simulink model "RLS_1a"  (R2023a)
settings: Solver=ode4  StartTime=0.0  StopTime=40  FixedStep=0.005  RelTol=1e-3
InitFcn:
  | RLS
values from neighbouring files (symbols this model uses):
  K_scheduled = zeros(length(V_op), 2)    [CAL3.m]    (also in CUB.m; DLC2.m; MUS.m; OHZ.m)
  V_op = 5:5:85    [CAL3.m]    (also in CUB.m; DLC2.m; MUS.m; OHZ.m)
  X_track = [linspace(0, runway_length, 200)'; runway_length + R_track * cos(theta_circ(2:end))]    [CAL3.m]    (also in CUB.m = [0; 5000]; DLC2.m = 0:0.1:total_track_length; MUS.m = [0; 2000]; OHZ.m = [0; 2000])
  Y_track = [zeros(200, 1); R_track + R_track * sin(theta_circ(2:end))]    [CAL3.m]    (also in CUB.m = [0; 0]; DLC2.m = zeros(size(X_track)); MUS.m = [0; 0]; OHZ.m = [0; 0])
libraries: simulink x2, slpidlib x1
(part 1 of 2)
settings Model: NumberOfSteps=1000  SnapshotBufferSize=1000  SnapshotInterval=1000  Creator=KBISWAS  LastModifiedBy=KBISWAS

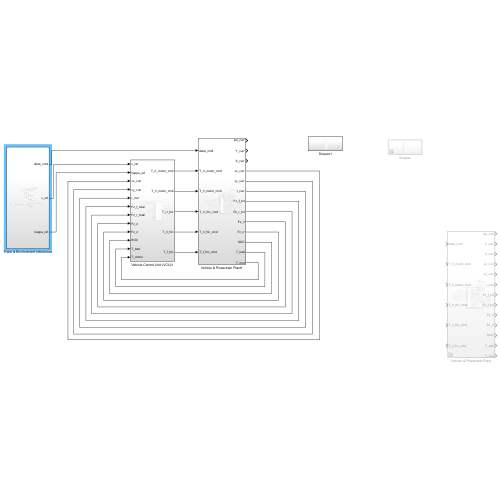
[thumbnail: Simulink's stored preview of the top-level diagram]
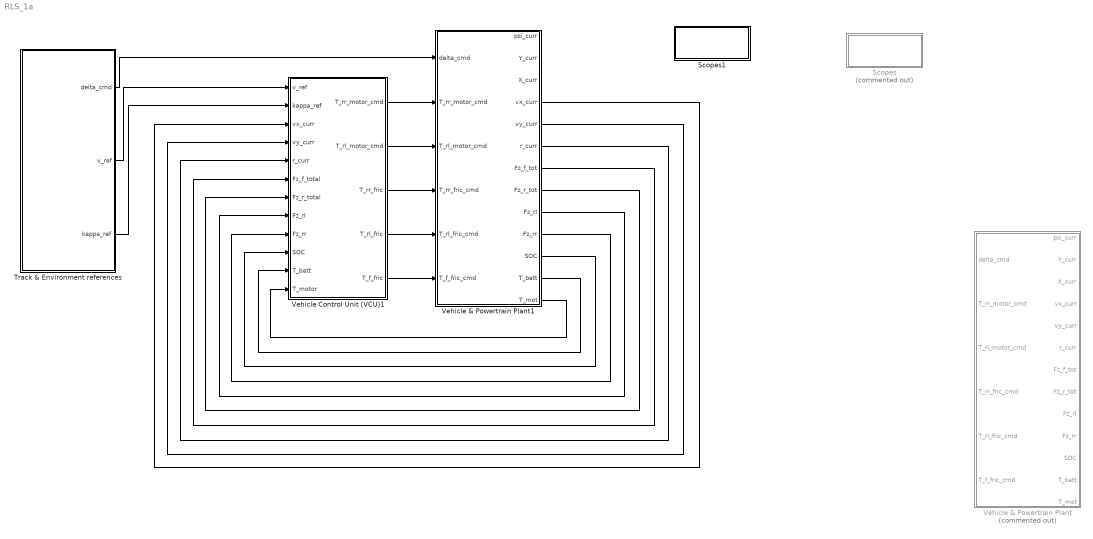
== system RLS_1a ==
  Scopes : Subsystem  Commented=on
  Scopes1 : Subsystem
  Track & Environment references : Subsystem
  Vehicle & Powertrain Plant : Subsystem  Commented=on
  Vehicle & Powertrain Plant1 : Subsystem
  Vehicle Control Unit (VCU)1 : Subsystem
  wires:
  Track & Environment references/2(v_ref) -> Vehicle Control Unit (VCU)1/1(v_ref)
  Vehicle Control Unit (VCU)1/1(T_rr_motor_cmd) -> Vehicle & Powertrain Plant1/2(T_rr_motor_cmd)
  Track & Environment references/3(kappa_ref) -> Vehicle Control Unit (VCU)1/2(kappa_ref)
  Track & Environment references/1(delta_cmd) -> Vehicle & Powertrain Plant1/1(delta_cmd)
  Vehicle Control Unit (VCU)1/2(T_rl_motor_cmd) -> Vehicle & Powertrain Plant1/3(T_rl_motor_cmd)
  Vehicle Control Unit (VCU)1/3(T_rr_fric) -> Vehicle & Powertrain Plant1/4(T_rr_fric_cmd)
  Vehicle Control Unit (VCU)1/4(T_rl_fric) -> Vehicle & Powertrain Plant1/5(T_rl_fric_cmd)
  Vehicle Control Unit (VCU)1/5(T_f_fric) -> Vehicle & Powertrain Plant1/6(T_f_fric_cmd)
  Vehicle & Powertrain Plant1/4(vx_curr) -> Vehicle Control Unit (VCU)1/3(vx_curr)
  Vehicle & Powertrain Plant1/5(vy_curr) -> Vehicle Control Unit (VCU)1/4(vy_curr)
  Vehicle & Powertrain Plant1/6(r_curr) -> Vehicle Control Unit (VCU)1/5(r_curr)
  Vehicle & Powertrain Plant1/7(Fz_f_tot) -> Vehicle Control Unit (VCU)1/6(Fz_f_total)
  Vehicle & Powertrain Plant1/8(Fz_r_tot) -> Vehicle Control Unit (VCU)1/7(Fz_r_total)
  Vehicle & Powertrain Plant1/9(Fz_rl) -> Vehicle Control Unit (VCU)1/8(Fz_rl)
  Vehicle & Powertrain Plant1/10(Fz_rr) -> Vehicle Control Unit (VCU)1/9(Fz_rr)
  Vehicle & Powertrain Plant1/11(SOC) -> Vehicle Control Unit (VCU)1/10(SOC)
  Vehicle & Powertrain Plant1/12(T_batt) -> Vehicle Control Unit (VCU)1/11(T_batt)
  Vehicle & Powertrain Plant1/13(T_mot) -> Vehicle Control Unit (VCU)1/12(T_motor)

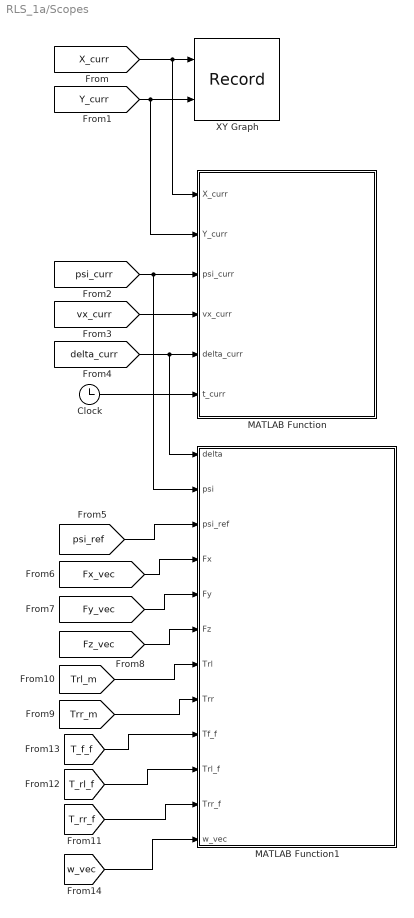
== system RLS_1a/Scopes ==
  Clock : Clock
  MATLAB Function : MATLAB Function  TreatAsAtomicUnit=on
  MATLAB Function1 : MATLAB Function  TreatAsAtomicUnit=on
  XY Graph : Record  FileSettingsInternal="{\"entries\":[{\"content\":{\"excelSettings\":{\"content\":{},\"type\":\"Streamout.ExcelSettings\"}},\"type\":\"Streamout.FileSettingStorage\",\"uuid\":\"\"}],\"packageUris\":[\"http:\\/\\/schema.mathworks.com\\/mf0\\/streamout_blocks\\/R2020a\"],\"version\":\"1.0\"}"  Layout=[1 1]  SignalsInternal="{\"entries\":[{\"content\":{},\"type\":\"RecordBlkView.InputSignals\",\"uuid\":\"\"}],\"packageUris\":[\"http:\\/\\/schema.mathworks.com\\/mf0\\/streamout_blocks\\/R2020a\"],\"version\":\"1.0\"}"  VisualizationBindings="{\"xyplotplugin\":{\"info\":[{\"series\":[],\"subplotID\":1}]}}"  CompatibilityTag=XY
  wires:
  [X_curr] -> MATLAB Function/1(X_curr), XY Graph/1
  [Y_curr] -> MATLAB Function/2(Y_curr), XY Graph/2
  [psi_curr] -> MATLAB Function/3(psi_curr), MATLAB Function1/2(psi)
  [vx_curr] -> MATLAB Function/4(vx_curr)
  [delta_curr] -> MATLAB Function1/1(delta), MATLAB Function/5(delta_curr)
  Clock/1 -> MATLAB Function/6(t_curr)
  [psi_ref] -> MATLAB Function1/3(psi_ref)
  [Fx_vec] -> MATLAB Function1/4(Fx)
  [Fy_vec] -> MATLAB Function1/5(Fy)
  [Fz_vec] -> MATLAB Function1/6(Fz)
  [Trr_m] -> MATLAB Function1/8(Trr)
  [Trl_m] -> MATLAB Function1/7(Trl)
  [T_f_f] -> MATLAB Function1/9(Tf_f)
  [T_rr_f] -> MATLAB Function1/11(Trr_f)
  [T_rl_f] -> MATLAB Function1/10(Trl_f)
  [w_vec] -> MATLAB Function1/12(w_vec)

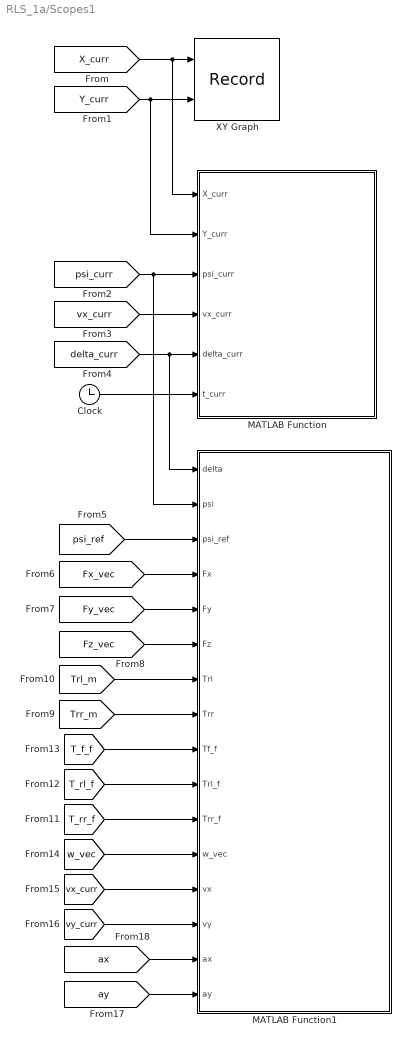
== system RLS_1a/Scopes1 ==
  Clock : Clock
  MATLAB Function : MATLAB Function  TreatAsAtomicUnit=on
  MATLAB Function1 : MATLAB Function  TreatAsAtomicUnit=on
  XY Graph : Record  FileSettingsInternal="{\"entries\":[{\"content\":{\"excelSettings\":{\"content\":{},\"type\":\"Streamout.ExcelSettings\"}},\"type\":\"Streamout.FileSettingStorage\",\"uuid\":\"\"}],\"packageUris\":[\"http:\\/\\/schema.mathworks.com\\/mf0\\/streamout_blocks\\/R2020a\"],\"version\":\"1.0\"}"  Layout=[1 1]  SignalsInternal="{\"entries\":[{\"content\":{\"signals\":[{\"content\":{\"blockPath\":[],\"dimensions\":[1],\"domain\":\"\",\"lineColor\":\"#a2142f\",\"plots\":[1],\"port\":1,\"sid\":[\"\"],\"signalID\":386165,\"signalName\":\"From\"},\"type\":\"RecordBlkView.Signal\",\"uuid\":\"\"},{\"content\":{\"blockPath\":[],\"dimensions\":[1],\"domain\":\"\",\"lineColor\":\"#139fff\",\"plots\":[1],\"port\":2,\"sid\":[\"\"],\"signalID\":386169,\"signalName\":\"From1\"},\"type\":\"RecordBlkView.Signal\",\"uuid\":\"\"}]},\"type\":\"RecordBlkView.InputSignals\",\"uuid\":\"\"}],\"packageUris\":[\"http:\\/\\/schema.mathworks.com\\/mf0\\/streamout_blocks\\/R2020a\"],\"version\":\"1.0\"}"  VisualizationBindings="{\"xyplotplugin\":{\"info\":[{\"series\":[{\"bindingParametersList\":[{\"parameter\":\"X-Axis\",\"signalID\":386165,\"signalName\":\"From\"},{\"parameter\":\"Y-Axis\",\"signalID\":386169,\"signalName\":\"From1\"}],\"seriesID\":29660}],\"subplotID\":1}]}}"  CompatibilityTag=XY
  wires:
  [X_curr] -> MATLAB Function/1(X_curr), XY Graph/1
  [Y_curr] -> MATLAB Function/2(Y_curr), XY Graph/2
  [psi_curr] -> MATLAB Function/3(psi_curr), MATLAB Function1/2(psi)
  [vx_curr] -> MATLAB Function/4(vx_curr)
  [delta_curr] -> MATLAB Function1/1(delta), MATLAB Function/5(delta_curr)
  Clock/1 -> MATLAB Function/6(t_curr)
  [psi_ref] -> MATLAB Function1/3(psi_ref)
  [Fx_vec] -> MATLAB Function1/4(Fx)
  [Fy_vec] -> MATLAB Function1/5(Fy)
  [Fz_vec] -> MATLAB Function1/6(Fz)
  [Trr_m] -> MATLAB Function1/8(Trr)
  [Trl_m] -> MATLAB Function1/7(Trl)
  [T_f_f] -> MATLAB Function1/9(Tf_f)
  [T_rr_f] -> MATLAB Function1/11(Trr_f)
  [T_rl_f] -> MATLAB Function1/10(Trl_f)
  [w_vec] -> MATLAB Function1/12(w_vec)
  [vx_curr] -> MATLAB Function1/13(vx)
  [vy_curr] -> MATLAB Function1/14(vy)
  [ax] -> MATLAB Function1/15(ax)
  [ay] -> MATLAB Function1/16(ay)

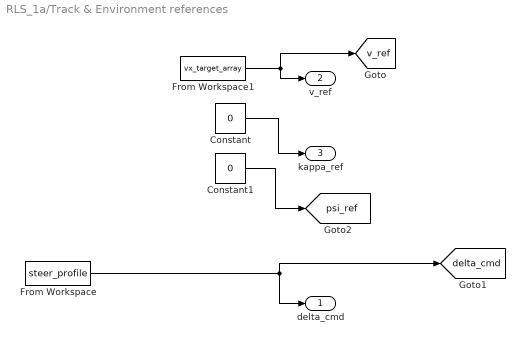
== system RLS_1a/Track & Environment references ==
  Constant : Constant  Value=0
  Constant1 : Constant  Value=0
  From Workspace : FromWorkspace  VariableName=steer_profile
  From Workspace1 : FromWorkspace  VariableName=vx_target_array
  delta_cmd : Outport
  v_ref : Outport  Port=2
  kappa_ref : Outport  Port=3
  tag scope: delta_cmd=global, psi_ref=global, v_ref=global
  wires:
  From Workspace/1 -> [delta_cmd], delta_cmd/1
  From Workspace1/1 -> v_ref/1, [v_ref]
  Constant1/1 -> [psi_ref]
  Constant/1 -> kappa_ref/1

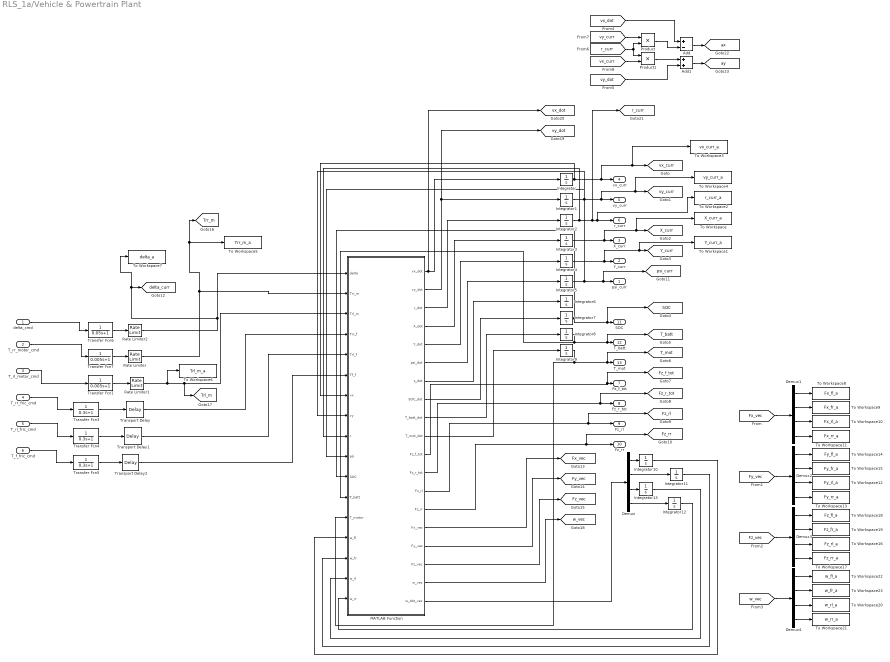
== system RLS_1a/Vehicle & Powertrain Plant ==
  delta_cmd : Inport
  T_rr_motor_cmd : Inport  Port=2
  T_rl_motor_cmd : Inport  Port=3
  T_rr_fric_cmd : Inport  Port=4
  T_rl_fric_cmd : Inport  Port=5
  T_f_fric_cmd : Inport  Port=6
  Add : Sum  Inputs=+-
  Add1 : Sum
  Demux{,1..4} (5 alike) : Demux
  Integrator : Integrator  InitialCondition=5
  Integrator{1..6,10..13} (10 alike) : Integrator
  Integrator7 : Integrator  InitialCondition=0.9
  Integrator8 : Integrator  InitialCondition=30
  Integrator9 : Integrator  InitialCondition=30
  MATLAB Function : MATLAB Function  TreatAsAtomicUnit=on
  Product : Product
  Product1 : Product
  Rate Limiter : RateLimiter  RisingSlewLimit=1500  FallingSlewLimit=-1500  SampleTimeMode=inherited
  Rate Limiter1 : RateLimiter  RisingSlewLimit=1500  FallingSlewLimit=-1500  SampleTimeMode=inherited
  Rate Limiter2 : RateLimiter  RisingSlewLimit=0.05  FallingSlewLimit=-0.05  SampleTimeMode=inherited
  To Workspace : ToWorkspace  VariableName=X_curr_a  SaveFormat=Timeseries  SampleTime=-1
  To Workspace1 : ToWorkspace  VariableName=Y_curr_a  SaveFormat=Timeseries  SampleTime=-1
  To Workspace10 : ToWorkspace  VariableName=Fx_rl_a  SaveFormat=Timeseries  SampleTime=-1
  To Workspace11 : ToWorkspace  VariableName=Fx_rr_a  SaveFormat=Timeseries  SampleTime=-1
  To Workspace12 : ToWorkspace  VariableName=Fy_rl_a  SaveFormat=Timeseries  SampleTime=-1
  To Workspace13 : ToWorkspace  VariableName=Fy_rr_a  SaveFormat=Timeseries  SampleTime=-1
  To Workspace14 : ToWorkspace  VariableName=Fy_fl_a  SaveFormat=Timeseries  SampleTime=-1
  To Workspace15 : ToWorkspace  VariableName=Fy_fr_a  SaveFormat=Timeseries  SampleTime=-1
  To Workspace16 : ToWorkspace  VariableName=Fz_rl_a  SaveFormat=Timeseries  SampleTime=-1
  To Workspace17 : ToWorkspace  VariableName=Fz_rr_a  SaveFormat=Timeseries  SampleTime=-1
  To Workspace18 : ToWorkspace  VariableName=Fz_fl_a  SaveFormat=Timeseries  SampleTime=-1
  To Workspace19 : ToWorkspace  VariableName=Fz_fr_a  SaveFormat=Timeseries  SampleTime=-1
  To Workspace2 : ToWorkspace  VariableName=r_curr_a  SaveFormat=Timeseries  SampleTime=-1
  To Workspace20 : ToWorkspace  VariableName=w_rl_a  SaveFormat=Timeseries  SampleTime=-1
  To Workspace21 : ToWorkspace  VariableName=w_rr_a  SaveFormat=Timeseries  SampleTime=-1
  To Workspace22 : ToWorkspace  VariableName=w_fl_a  SaveFormat=Timeseries  SampleTime=-1
  To Workspace23 : ToWorkspace  VariableName=w_fr_a  SaveFormat=Timeseries  SampleTime=-1
  To Workspace3 : ToWorkspace  VariableName=vx_curr_a  SaveFormat=Timeseries  SampleTime=-1
  To Workspace4 : ToWorkspace  VariableName=vy_curr_a  SaveFormat=Timeseries  SampleTime=-1
  To Workspace5 : ToWorkspace  VariableName=Trr_m_a  SaveFormat=Timeseries  SampleTime=-1
  To Workspace6 : ToWorkspace  VariableName=Trl_m_a  SaveFormat=Timeseries  SampleTime=-1
  To Workspace7 : ToWorkspace  VariableName=delta_a  SaveFormat=Timeseries  SampleTime=-1
  To Workspace8 : ToWorkspace  VariableName=Fx_fl_a  SaveFormat=Timeseries  SampleTime=-1
  To Workspace9 : ToWorkspace  VariableName=Fx_fr_a  SaveFormat=Timeseries  SampleTime=-1
  Transfer Fcn1 : TransferFcn  Denominator=[0.005 1]
  Transfer Fcn3 : TransferFcn  Denominator=[0.3 1]
  Transfer Fcn4 : TransferFcn  Denominator=[0.3 1]
  Transfer Fcn5 : TransferFcn  Denominator=[0.3 1]
  Transfer Fcn6 : TransferFcn  Numerator=1  Denominator=[0.05 1]
  Transfer Fcn7 : TransferFcn  Denominator=[0.005 1]
  Transport Delay : TransportDelay  DelayTime=0.03
  Transport Delay1 : TransportDelay  DelayTime=0.03
  Transport Delay2 : TransportDelay  DelayTime=0.03
  psi_curr : Outport
  Y_curr : Outport  Port=2
  X_curr : Outport  Port=3
  vx_curr : Outport  Port=4
  vy_curr : Outport  Port=5
  r_curr : Outport  Port=6
  Fz_f_tot : Outport  Port=7
  Fz_r_tot : Outport  Port=8
  Fz_rl : Outport  Port=9
  Fz_rr : Outport  Port=10
  SOC : Outport  Port=11
  T_batt : Outport  Port=12
  T_mot : Outport  Port=13
  tag scope: Fx_vec=global, Fy_vec=global, Fz_f_tot=global, Fz_r_tot=global, Fz_rl=global, Fz_rr=global, Fz_vec=global, SOC=global, T_batt=global, T_mot=global, Trl_m=global, Trr_m=global, X_curr=global, Y_curr=global, ax=global, ay=global, delta_curr=global, psi_curr=global, r_curr=global, vx_curr=global, vx_dot=global, vy_curr=global, vy_dot=global, w_vec=global
  wires:
  delta_cmd/1 -> Transfer Fcn6/1
  T_rr_motor_cmd/1 -> Transfer Fcn7/1
  T_rl_motor_cmd/1 -> Transfer Fcn1/1
  T_rr_fric_cmd/1 -> Transfer Fcn3/1
  T_rl_fric_cmd/1 -> Transfer Fcn4/1
  T_f_fric_cmd/1 -> Transfer Fcn5/1
  Rate Limiter2/1 -> MATLAB Function/1(delta), To Workspace7/1, [delta_curr]
  Rate Limiter/1 -> MATLAB Function/2(Trr_m), To Workspace5/1, [Trr_m]
  Rate Limiter1/1 -> To Workspace6/1, MATLAB Function/3(Trl_m), [Trl_m]
  Transport Delay/1 -> MATLAB Function/4(Trr_f)
  Transport Delay1/1 -> MATLAB Function/5(Trl_f)
  Transport Delay2/1 -> MATLAB Function/6(Tf_f)
  MATLAB Function/3(r_dot) -> Integrator2/1
  MATLAB Function/4(X_dot) -> Integrator3/1
  MATLAB Function/5(Y_dot) -> Integrator4/1
  MATLAB Function/6(psi_dot) -> Integrator5/1
  MATLAB Function/7(s_dot) -> Integrator6/1
  MATLAB Function/8(SOC_dot) -> Integrator7/1
  Integrator/1 -> MATLAB Function/7(vx), To Workspace3/1, [vx_curr], vx_curr/1
  Integrator1/1 -> MATLAB Function/8(vy), To Workspace4/1, [vy_curr], vy_curr/1
  Integrator5/1 -> MATLAB Function/10(psi), [psi_curr], psi_curr/1
  Integrator8/1 -> MATLAB Function/12(T_batt), [T_batt], T_batt/1
  Integrator9/1 -> MATLAB Function/13(T_motor), [T_mot], T_mot/1
  Integrator4/1 -> To Workspace1/1, [Y_curr], Y_curr/1
  Integrator3/1 -> To Workspace/1, [X_curr], X_curr/1
  MATLAB Function/11(Fz_f_tot) -> [Fz_f_tot], Fz_f_tot/1
  Integrator7/1 -> MATLAB Function/11(SOC), [SOC], SOC/1
  MATLAB Function/14(Fz_rr) -> [Fz_rr], Fz_rr/1
  MATLAB Function/15(Fx_vec) -> [Fx_vec]
  MATLAB Function/17(Fz_vec) -> [Fz_vec]
  MATLAB Function/9(T_batt_dot) -> Integrator8/1
  MATLAB Function/10(T_mot_dot) -> Integrator9/1
  MATLAB Function/12(Fz_r_tot) -> [Fz_r_tot], Fz_r_tot/1
  MATLAB Function/13(Fz_rl) -> [Fz_rl], Fz_rl/1
  MATLAB Function/16(Fy_vec) -> [Fy_vec]
  MATLAB Function/18(w_vec) -> [w_vec]
  Demux/4 -> Integrator12/1
  Demux/3 -> Integrator13/1
  Demux/2 -> Integrator11/1
  Demux/1 -> Integrator10/1
  MATLAB Function/19(w_dot_vec) -> Demux/1
  Integrator10/1 -> MATLAB Function/14(w_fl)
  Integrator11/1 -> MATLAB Function/15(w_fr)
  Integrator12/1 -> MATLAB Function/17(w_rr)
  Integrator13/1 -> MATLAB Function/16(w_rl)
  Transfer Fcn6/1 -> Rate Limiter2/1
  Transfer Fcn7/1 -> Rate Limiter/1
  Transfer Fcn1/1 -> Rate Limiter1/1
  Transfer Fcn4/1 -> Transport Delay1/1
  Transfer Fcn5/1 -> Transport Delay2/1
  Transfer Fcn3/1 -> Transport Delay/1
  [vx_dot] -> Add/1
  Product/1 -> Add/2
  MATLAB Function/2(vy_dot) -> [vy_dot], Integrator1/1
  Add1/1 -> [ay]
  MATLAB Function/1(vx_dot) -> [vx_dot], Integrator/1
  [vy_curr] -> Product/1
  Integrator2/1 -> [r_curr], To Workspace2/1, r_curr/1, MATLAB Function/9(r)
  [vy_dot] -> Add1/2
  [vx_curr] -> Product1/2
  [r_curr] -> Product1/1, Product/2
  Product1/1 -> Add1/1
  Add/1 -> [ax]
  Demux4/4 -> To Workspace21/1
  Demux4/3 -> To Workspace20/1
  Demux4/1 -> To Workspace22/1
  Demux4/2 -> To Workspace23/1
  [Fy_vec] -> Demux2/1
  [Fz_vec] -> Demux3/1
  [Fx_vec] -> Demux1/1
  Demux3/4 -> To Workspace17/1
  Demux2/2 -> To Workspace15/1
  Demux3/2 -> To Workspace19/1
  Demux3/1 -> To Workspace18/1
  Demux2/1 -> To Workspace14/1
  Demux1/3 -> To Workspace10/1
  Demux1/4 -> To Workspace11/1
  Demux1/2 -> To Workspace9/1
  Demux3/3 -> To Workspace16/1
  Demux2/3 -> To Workspace12/1
  Demux2/4 -> To Workspace13/1
  Demux1/1 -> To Workspace8/1
  [w_vec] -> Demux4/1

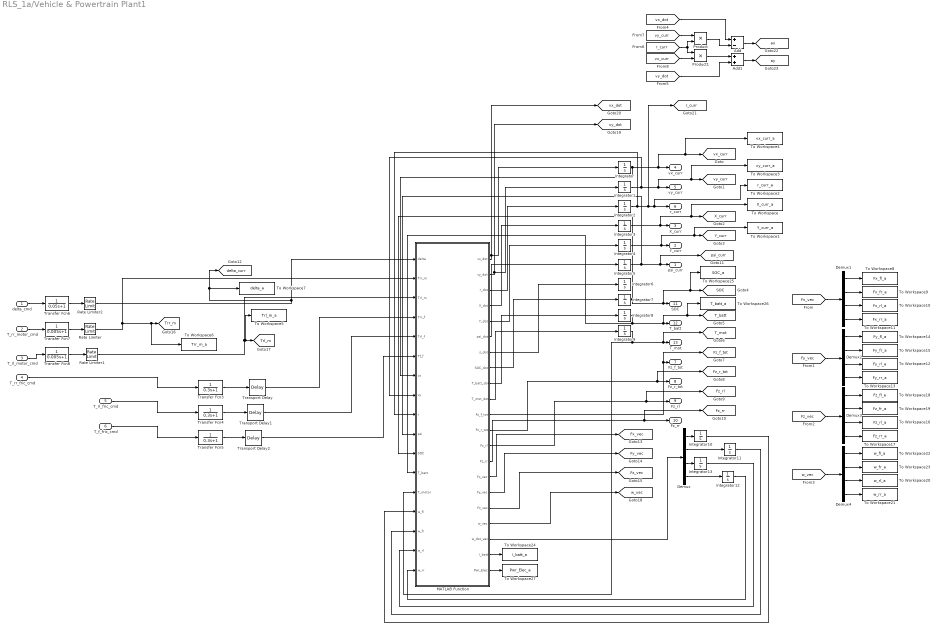
== system RLS_1a/Vehicle & Powertrain Plant1 ==
  delta_cmd : Inport
  T_rr_motor_cmd : Inport  Port=2
  T_rl_motor_cmd : Inport  Port=3
  T_rr_fric_cmd : Inport  Port=4
  T_rl_fric_cmd : Inport  Port=5
  T_f_fric_cmd : Inport  Port=6
  Add : Sum  Inputs=+-
  Add1 : Sum
  Demux{,1..4} (5 alike) : Demux
  Integrator : Integrator  InitialCondition=5
  Integrator{1..6,10..13} (10 alike) : Integrator
  Integrator7 : Integrator  InitialCondition=0.9
  Integrator8 : Integrator  InitialCondition=30
  Integrator9 : Integrator  InitialCondition=30
  MATLAB Function : MATLAB Function  TreatAsAtomicUnit=on
  Product : Product
  Product1 : Product
  Rate Limiter : RateLimiter  RisingSlewLimit=500  FallingSlewLimit=-500  SampleTimeMode=inherited
  Rate Limiter1 : RateLimiter  RisingSlewLimit=500  FallingSlewLimit=-500  SampleTimeMode=inherited
  Rate Limiter2 : RateLimiter  RisingSlewLimit=10  FallingSlewLimit=-10  SampleTimeMode=inherited
  To Workspace : ToWorkspace  VariableName=X_curr_a  SaveFormat=Timeseries  SampleTime=-1
  To Workspace1 : ToWorkspace  VariableName=Y_curr_a  SaveFormat=Timeseries  SampleTime=-1
  To Workspace10 : ToWorkspace  VariableName=Fx_rl_a  SaveFormat=Timeseries  SampleTime=-1
  To Workspace11 : ToWorkspace  VariableName=Fx_rr_a  SaveFormat=Timeseries  SampleTime=-1
  To Workspace12 : ToWorkspace  VariableName=Fy_rl_a  SaveFormat=Timeseries  SampleTime=-1
  To Workspace13 : ToWorkspace  VariableName=Fy_rr_a  SaveFormat=Timeseries  SampleTime=-1
  To Workspace14 : ToWorkspace  VariableName=Fy_fl_a  SaveFormat=Timeseries  SampleTime=-1
  To Workspace15 : ToWorkspace  VariableName=Fy_fr_a  SaveFormat=Timeseries  SampleTime=-1
  To Workspace16 : ToWorkspace  VariableName=Fz_rl_a  SaveFormat=Timeseries  SampleTime=-1
  To Workspace17 : ToWorkspace  VariableName=Fz_rr_a  SaveFormat=Timeseries  SampleTime=-1
  To Workspace18 : ToWorkspace  VariableName=Fz_fl_a  SaveFormat=Timeseries  SampleTime=-1
  To Workspace19 : ToWorkspace  VariableName=Fz_fr_a  SaveFormat=Timeseries  SampleTime=-1
  To Workspace2 : ToWorkspace  VariableName=r_curr_a  SaveFormat=Timeseries  SampleTime=-1
  To Workspace20 : ToWorkspace  VariableName=w_rl_a  SaveFormat=Timeseries  SampleTime=-1
  To Workspace21 : ToWorkspace  VariableName=w_rr_a  SaveFormat=Timeseries  SampleTime=-1
  To Workspace22 : ToWorkspace  VariableName=w_fl_a  SaveFormat=Timeseries  SampleTime=-1
  To Workspace23 : ToWorkspace  VariableName=w_fr_a  SaveFormat=Timeseries  SampleTime=-1
  To Workspace24 : ToWorkspace  VariableName=I_batt_a  SaveFormat=Timeseries  SampleTime=-1
  To Workspace25 : ToWorkspace  VariableName=SOC_a  SaveFormat=Timeseries  SampleTime=-1
  To Workspace26 : ToWorkspace  VariableName=T_batt_a  SaveFormat=Timeseries  SampleTime=-1
  To Workspace27 : ToWorkspace  VariableName=Pwr_Elec_a  SaveFormat=Timeseries  SampleTime=-1
  To Workspace3 : ToWorkspace  VariableName=vy_curr_a  SaveFormat=Timeseries  SampleTime=-1
  To Workspace4 : ToWorkspace  VariableName=vx_curr_a  SaveFormat=Timeseries  SampleTime=-1
  To Workspace5 : ToWorkspace  VariableName=Trl_m_a  SaveFormat=Timeseries  SampleTime=-1
  To Workspace6 : ToWorkspace  VariableName=Trr_m_a  SaveFormat=Timeseries  SampleTime=-1
  To Workspace7 : ToWorkspace  VariableName=delta_a  SaveFormat=Timeseries  SampleTime=-1
  To Workspace8 : ToWorkspace  VariableName=Fx_fl_a  SaveFormat=Timeseries  SampleTime=-1
  To Workspace9 : ToWorkspace  VariableName=Fx_fr_a  SaveFormat=Timeseries  SampleTime=-1
  Transfer Fcn3 : TransferFcn  Denominator=[0.3 1]
  Transfer Fcn4 : TransferFcn  Denominator=[0.3 1]
  Transfer Fcn5 : TransferFcn  Denominator=[0.3 1]
  Transfer Fcn6 : TransferFcn  Numerator=1  Denominator=[0.05 1]
  Transfer Fcn7 : TransferFcn  Denominator=[0.005 1]
  Transfer Fcn8 : TransferFcn  Denominator=[0.005 1]
  Transport Delay : TransportDelay  DelayTime=0.03
  Transport Delay1 : TransportDelay  DelayTime=0.03
  Transport Delay2 : TransportDelay  DelayTime=0.03
  psi_curr : Outport
  Y_curr : Outport  Port=2
  X_curr : Outport  Port=3
  vx_curr : Outport  Port=4
  vy_curr : Outport  Port=5
  r_curr : Outport  Port=6
  Fz_f_tot : Outport  Port=7
  Fz_r_tot : Outport  Port=8
  Fz_rl : Outport  Port=9
  Fz_rr : Outport  Port=10
  SOC : Outport  Port=11
  T_batt : Outport  Port=12
  T_mot : Outport  Port=13
  tag scope: Fx_vec=global, Fy_vec=global, Fz_f_tot=global, Fz_r_tot=global, Fz_rl=global, Fz_rr=global, Fz_vec=global, SOC=global, T_batt=global, T_mot=global, Trl_m=global, Trr_m=global, X_curr=global, Y_curr=global, ax=global, ay=global, delta_curr=global, psi_curr=global, r_curr=global, vx_curr=global, vx_dot=global, vy_curr=global, vy_dot=global, w_vec=global
  wires:
  delta_cmd/1 -> Transfer Fcn6/1
  T_rr_fric_cmd/1 -> Transfer Fcn3/1
  T_rl_fric_cmd/1 -> Transfer Fcn4/1
  T_f_fric_cmd/1 -> Transfer Fcn5/1
  Transfer Fcn6/1 -> Rate Limiter2/1
  Rate Limiter/1 -> MATLAB Function/2(Trr_m), To Workspace6/1, [Trr_m]
  Rate Limiter1/1 -> MATLAB Function/3(Trl_m), To Workspace5/1, [Trl_m]
  Transfer Fcn3/1 -> Transport Delay/1
  Transfer Fcn4/1 -> Transport Delay1/1
  Transfer Fcn5/1 -> Transport Delay2/1
  MATLAB Function/1(vx_dot) -> [vx_dot], Integrator/1
  MATLAB Function/2(vy_dot) -> [vy_dot], Integrator1/1
  MATLAB Function/3(r_dot) -> Integrator2/1
  MATLAB Function/4(X_dot) -> Integrator3/1
  MATLAB Function/5(Y_dot) -> Integrator4/1
  MATLAB Function/6(psi_dot) -> Integrator5/1
  MATLAB Function/7(s_dot) -> Integrator6/1
  MATLAB Function/8(SOC_dot) -> Integrator7/1
  Integrator/1 -> MATLAB Function/7(vx), To Workspace4/1, [vx_curr], vx_curr/1
  Integrator1/1 -> MATLAB Function/8(vy), To Workspace3/1, [vy_curr], vy_curr/1
  Integrator2/1 -> [r_curr], To Workspace2/1, r_curr/1, MATLAB Function/9(r)
  Integrator5/1 -> MATLAB Function/10(psi), [psi_curr], psi_curr/1
  Integrator8/1 -> MATLAB Function/12(T_batt), To Workspace26/1, [T_batt], T_batt/1
  Integrator9/1 -> MATLAB Function/13(T_motor), [T_mot], T_mot/1
  Integrator4/1 -> To Workspace1/1, [Y_curr], Y_curr/1
  Integrator3/1 -> To Workspace/1, [X_curr], X_curr/1
  MATLAB Function/11(Fz_f_tot) -> [Fz_f_tot], Fz_f_tot/1
  Integrator7/1 -> MATLAB Function/11(SOC), To Workspace25/1, [SOC], SOC/1
  MATLAB Function/14(Fz_rr) -> [Fz_rr], Fz_rr/1
  MATLAB Function/15(Fx_vec) -> [Fx_vec]
  MATLAB Function/17(Fz_vec) -> [Fz_vec]
  MATLAB Function/9(T_batt_dot) -> Integrator8/1
  MATLAB Function/10(T_mot_dot) -> Integrator9/1
  MATLAB Function/12(Fz_r_tot) -> [Fz_r_tot], Fz_r_tot/1
  MATLAB Function/13(Fz_rl) -> [Fz_rl], Fz_rl/1
  MATLAB Function/16(Fy_vec) -> [Fy_vec]
  MATLAB Function/18(w_vec) -> [w_vec]
  Demux/4 -> Integrator12/1
  Demux/3 -> Integrator13/1
  Demux/2 -> Integrator11/1
  Demux/1 -> Integrator10/1
  MATLAB Function/19(w_dot_vec) -> Demux/1
  Integrator10/1 -> MATLAB Function/14(w_fl)
  Integrator11/1 -> MATLAB Function/15(w_fr)
  Integrator12/1 -> MATLAB Function/17(w_rr)
  Integrator13/1 -> MATLAB Function/16(w_rl)
  T_rr_motor_cmd/1 -> Transfer Fcn7/1
  Transfer Fcn7/1 -> Rate Limiter/1
  Transfer Fcn8/1 -> Rate Limiter1/1
  T_rl_motor_cmd/1 -> Transfer Fcn8/1
  [Fx_vec] -> Demux1/1
  Demux1/1 -> To Workspace8/1
  Demux1/2 -> To Workspace9/1
  Demux1/3 -> To Workspace10/1
  Demux1/4 -> To Workspace11/1
  Demux2/2 -> To Workspace15/1
  Demux2/4 -> To Workspace13/1
  Demux2/1 -> To Workspace14/1
  [Fy_vec] -> Demux2/1
  Demux2/3 -> To Workspace12/1
  [Fz_vec] -> Demux3/1
  Demux3/1 -> To Workspace18/1
  Demux3/3 -> To Workspace16/1
  Demux3/4 -> To Workspace17/1
  Demux3/2 -> To Workspace19/1
  Demux4/2 -> To Workspace23/1
  Demux4/4 -> To Workspace21/1
  Demux4/1 -> To Workspace22/1
  Demux4/3 -> To Workspace20/1
  [w_vec] -> Demux4/1
  [vy_curr] -> Product/1
  [r_curr] -> Product1/1, Product/2
  Product/1 -> Add/2
  [vx_dot] -> Add/1
  [vx_curr] -> Product1/2
  Product1/1 -> Add1/1
  [vy_dot] -> Add1/2
  Add/1 -> [ax]
  Add1/1 -> [ay]
  MATLAB Function/20(I_batt) -> To Workspace24/1
  MATLAB Function/21(Pwr_Elec) -> To Workspace27/1
  Rate Limiter2/1 -> MATLAB Function/1(delta), To Workspace7/1, [delta_curr]
  Transport Delay/1 -> MATLAB Function/4(Trr_f)
  Transport Delay1/1 -> MATLAB Function/5(Trl_f)
  Transport Delay2/1 -> MATLAB Function/6(Tf_f)

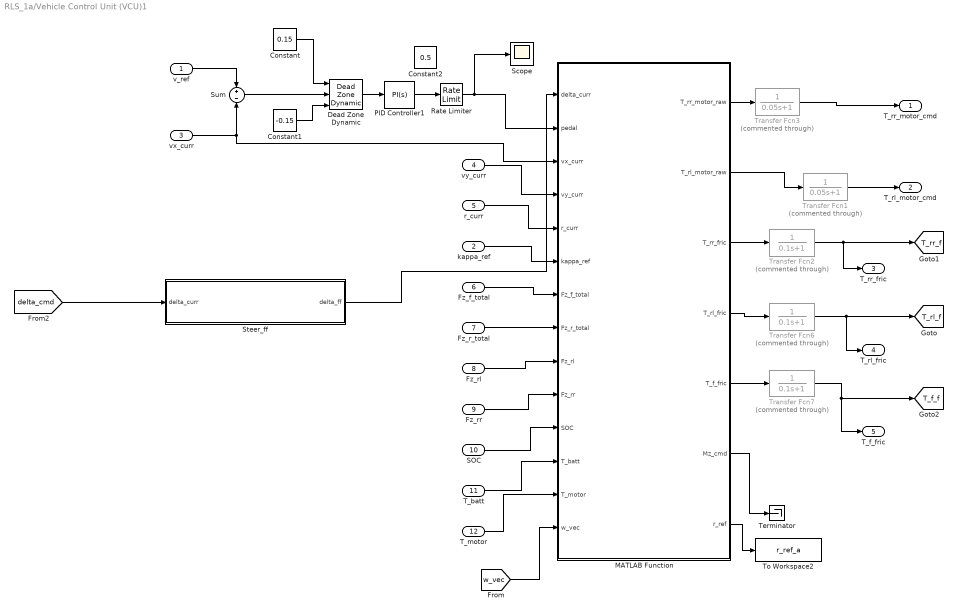
== system RLS_1a/Vehicle Control Unit (VCU)1 ==
  v_ref : Inport
  kappa_ref : Inport  Port=2
  vx_curr : Inport  Port=3
  vy_curr : Inport  Port=4
  r_curr : Inport  Port=5
  Fz_f_total : Inport  Port=6
  Fz_r_total : Inport  Port=7
  Fz_rl : Inport  Port=8
  Fz_rr : Inport  Port=9
  SOC : Inport  Port=10
  T_batt : Inport  Port=11
  T_motor : Inport  Port=12
  Constant : Constant  Value=0.15
  Constant1 : Constant  Value=-0.15
  Constant2 : Constant  Value=0.5
  Dead Zone Dynamic : simulink/Discontinuities/Dead Zone Dynamic
  MATLAB Function : MATLAB Function  TreatAsAtomicUnit=on
  PID Controller1 : slpidlib/PID Controller  Controller=PI  Form=Parallel  TimeDomain=Continuous-time  UseExternalTs=off  SampleTime=-1  IntegratorMethod=Forward Euler  FilterMethod=Forward Euler  ControllerParametersSource=internal  P=0.2  I=0.5  UseKiTs=off  D=0  N=100  UseFilter=on  TunerSelectOption=Transfer Function Based (PID Tuner App)  InitialConditionSource=internal  InitialConditionForIntegrator=0  InitialConditionForFilter=0  DifferentiatorICPrevScaledInput=0  ExternalReset=none  TrackingMode=off  Kt=1  LimitOutput=on  SatLimitsSource=internal  UpperSaturationLimit=1  LowerSaturationLimit=-1  LinearizeAsGain=on  AntiWindupMode=clamping  Kb=1  LimitIntegrator=off  UpperIntegratorSaturationLimit=inf  LowerIntegratorSaturationLimit=-inf  POutMin=[]  POutMax=[]  IOutMin=[]  IOutMax=[]  DOutMin=[]  DOutMax=[]  NOutMin=[]  NOutMax=[]  SumOutMin=[]  SumOutMax=[]  SaturationOutMin=[]  SaturationOutMax=[]  PParamMin=[]  PParamMax=[]  IParamMin=[]  IParamMax=[]  DParamMin=[]  DParamMax=[]  NParamMin=[]  NParamMax=[]  KbParamMin=[]  KbParamMax=[]  KtParamMin=[]  KtParamMax=[]  KbOutMin=[]  KbOutMax=[]  KtOutMin=[]  KtOutMax=[]  IntegratorOutMin=[]  IntegratorOutMax=[]  FilterOutMin=[]  FilterOutMax=[]  SumI1OutMin=[]  SumI1OutMax=[]  SumI2OutMin=[]  SumI2OutMax=[]  SumI3OutMin=[]  SumI3OutMax=[]  SumI4OutMin=[]  SumI4OutMax=[]  SumDOutMin=[]  SumDOutMax=[]  DifferentiatorOutMin=[]  DifferentiatorOutMax=[]  FilterDiffOutCoefMin=[]  FilterDiffOutCoefMax=[]  ReciprocalOutMin=[]  ReciprocalOutMax=[]  SumDenOutMin=[]  SumDenOutMax=[]  SumNumOutMin=[]  SumNumOutMax=[]  DivideOutMin=[]  DivideOutMax=[]  UdiffTsProdOutMin=[]  UdiffTsProdOutMax=[]  NTsProdOutMin=[]  NTsProdOutMax=[]  UintegralTsProdOutMin=[]  UintegralTsProdOutMax=[]  UngainTsProdOutMin=[]  UngainTsProdOutMax=[]  ClampingZeroOutDataTypeStr=Inherit: Inherit via back propagation  ClampingZeroOutMin=[]  ClampingZeroOutMax=[]  FilterDenConstantOutDataTypeStr=Inherit: Inherit via back propagation  FilterDenConstantOutMin=[]  FilterDenConstantOutMax=[]  PCopyOutDataTypeStr=Inherit: Inherit via back propagation  PCopyOutMin=[]  PCopyOutMax=[]  NCopyOutDataTypeStr=Inherit: Inherit via back propagation  NCopyOutMin=[]  NCopyOutMax=[]  IntegratorContinuousStateAttributes=''  IntegratorStateMustResolveToSignalObject=off  IntegratorRTWStateStorageClass=Auto  FilterContinuousStateAttributes=''  FilterStateMustResolveToSignalObject=off  FilterRTWStateStorageClass=Auto  ParallelPVariant=InternalParameters  IdealPVariant=Disabled  IVariant=InternalParameters  DVariant=Disabled  IntegratorVariant=Continuous  SatVariant=Enabled  AWVariant=ContClampingParallel  PCopyVariant=Disabled  TRVariant=Disabled  FdbkBlocksVariant=Forward  IdealPFdbkVariant=Disabled  SatFdbkVariant=Disabled  DerivativeFilterVariant=Disabled  NVariant=Disabled  NCopyVariant=Disabled_SignalSpec  FilterICVariant=Disabled  IntegratorICVariant=InternalICs  ExternalResetVariant=Disabled  TRSumVariant=Passthrough  SumFdbkVariant=Disabled  SumVariant=Sum_PI  TsampFilterVariant=InternalTs  TsampNgainVariant=Passthrough  TsampIntegralVariant=Disabled_SignalSpec  ExternalSaturationOutDataTypeStr=Inherit: Same as second input
  Rate Limiter : RateLimiter  RisingSlewLimit=0.5  FallingSlewLimit=-4  SampleTimeMode=inherited
  Scope : Scope
  Steer_ff : Subsystem
  Sum : Sum  Inputs=+-
  Terminator : Terminator
  To Workspace2 : ToWorkspace  VariableName=r_ref_a  SaveFormat=Timeseries  SampleTime=-1
  Transfer Fcn1 : TransferFcn  Commented=through  Denominator=[0.05 1]
  Transfer Fcn2 : TransferFcn  Commented=through  Denominator=[0.1 1]
  Transfer Fcn3 : TransferFcn  Commented=through  Denominator=[0.05 1]
  Transfer Fcn6 : TransferFcn  Commented=through  Denominator=[0.1 1]
  Transfer Fcn7 : TransferFcn  Commented=through  Denominator=[0.1 1]
  T_rr_motor_cmd : Outport
  T_rl_motor_cmd : Outport  Port=2
  T_rr_fric : Outport  Port=3
  T_rl_fric : Outport  Port=4
  T_f_fric : Outport  Port=5
  tag scope: T_f_f=global, T_rl_f=global, T_rr_f=global
  wires:
  v_ref/1 -> Sum/1
  vy_curr/1 -> MATLAB Function/4(vy_curr)
  r_curr/1 -> MATLAB Function/5(r_curr)
  kappa_ref/1 -> MATLAB Function/6(kappa_ref)
  Fz_f_total/1 -> MATLAB Function/7(Fz_f_total)
  Fz_r_total/1 -> MATLAB Function/8(Fz_r_total)
  Fz_rl/1 -> MATLAB Function/9(Fz_rl)
  Fz_rr/1 -> MATLAB Function/10(Fz_rr)
  SOC/1 -> MATLAB Function/11(SOC)
  T_batt/1 -> MATLAB Function/12(T_batt)
  T_motor/1 -> MATLAB Function/13(T_motor)
  Rate Limiter/1 -> Scope/1, MATLAB Function/2(pedal)
  MATLAB Function/1(T_rr_motor_raw) -> Transfer Fcn3/1
  MATLAB Function/2(T_rl_motor_raw) -> Transfer Fcn1/1
  MATLAB Function/3(T_rr_fric) -> Transfer Fcn2/1
  MATLAB Function/4(T_rl_fric) -> Transfer Fcn6/1
  MATLAB Function/5(T_f_fric) -> Transfer Fcn7/1
  MATLAB Function/6(Mz_cmd) -> Terminator/1
  [w_vec] -> MATLAB Function/14(w_vec)
  MATLAB Function/7(r_ref) -> To Workspace2/1
  Steer_ff/1(delta_ff) -> MATLAB Function/1(delta_curr)
  [delta_cmd] -> Steer_ff/1(delta_curr)
  Transfer Fcn3/1 -> T_rr_motor_cmd/1
  Transfer Fcn1/1 -> T_rl_motor_cmd/1
  Transfer Fcn2/1 -> T_rr_fric/1, [T_rr_f]
  Transfer Fcn6/1 -> T_rl_fric/1, [T_rl_f]
  Transfer Fcn7/1 -> T_f_fric/1, [T_f_f]
  Dead Zone Dynamic/1 -> PID Controller1/1
  Constant/1 -> Dead Zone Dynamic/1
  Sum/1 -> Dead Zone Dynamic/2
  Constant1/1 -> Dead Zone Dynamic/3
  vx_curr/1 -> MATLAB Function/3(vx_curr), Sum/2
  PID Controller1/1 -> Rate Limiter/1

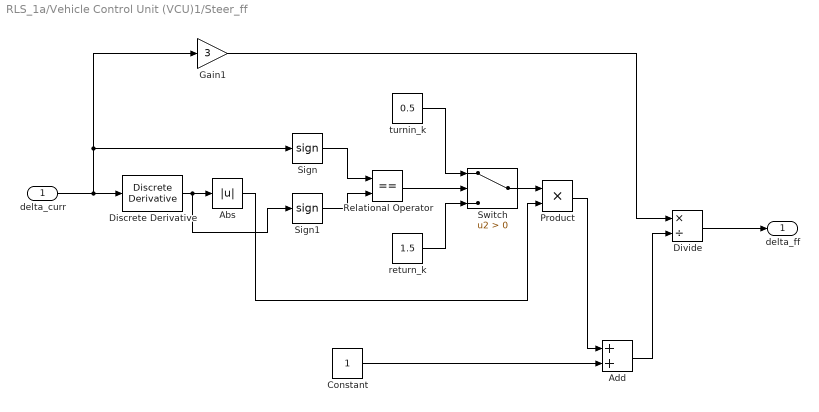
== system RLS_1a/Vehicle Control Unit (VCU)1/Steer_ff ==
  delta_curr : Inport
  Abs : Abs  SaturateOnIntegerOverflow=off
  Add : Sum
  Constant : Constant
  Discrete Derivative : simulink/Discrete/Discrete Derivative  gainval=1.0  ICPrevScaledInput=0.0  OutMin=[]  OutMax=[]  OutDataType=fixdt(1, 16)  OutScaling=2^-10  DoSatur=off
  Divide : Product  Inputs=*/
  Gain1 : Gain  Gain=3
  Product : Product
  Relational Operator : RelationalOperator  Operator===  OutDataTypeStr=boolean  RndMeth=Simplest  InputSameDT=off
  Sign : Signum
  Sign1 : Signum
  Switch : Switch  Criteria=u2 > Threshold  SaturateOnIntegerOverflow=off  InputSameDT=off
  return_k : Constant  Value=1.5
  turnin_k : Constant  Value=0.5
  delta_ff : Outport
  wires:
  Gain1/1 -> Divide/1
  return_k/1 -> Switch/3
  Switch/1 -> Product/1
  Product/1 -> Add/1
  Sign/1 -> Relational Operator/1
  delta_curr/1 -> Discrete Derivative/1, Gain1/1, Sign/1
  Relational Operator/1 -> Switch/2
  Add/1 -> Divide/2
  Discrete Derivative/1 -> Sign1/1, Abs/1
  Abs/1 -> Product/2
  Constant/1 -> Add/2
  Sign1/1 -> Relational Operator/2
  Divide/1 -> delta_ff/1
  turnin_k/1 -> Switch/1

== matlab function RLS_1a/Vehicle & Powertrain Plant/MATLAB Function ==
  data: delta input; Trr_m input; Trl_m input; Trr_f input; Trl_f input; Tf_f input; vx input; vy input; r input; psi input; SOC input; T_batt input; T_motor input; w_fl input; w_fr input; w_rl input; w_rr input; vx_dot output; vy_dot output; r_dot output; X_dot output; Y_dot output; psi_dot output; s_dot output; SOC_dot output; T_batt_dot output; T_mot_dot output; Fz_f_tot output; Fz_r_tot output; Fz_rl output; Fz_rr output; Fx_vec output; Fy_vec output; Fz_vec output; w_vec output; w_dot_vec output; veh_params parameter
function [vx_dot, vy_dot, r_dot, X_dot, Y_dot, psi_dot, s_dot, SOC_dot, T_batt_dot, T_mot_dot, Fz_f_tot, Fz_r_tot, Fz_rl, Fz_rr, Fx_vec, Fy_vec, Fz_vec, w_vec, w_dot_vec] = vehicle_physics_engine(delta, Trr_m, Trl_m, Trr_f, Trl_f, Tf_f, vx, vy, r, psi, SOC, T_batt, T_motor, w_fl, w_fr, w_rl, w_rr, veh_params)
    % =========================================================================
    % STABLE BASELINE 7-DOF PLANAR PHYSICS (Zero Roll/Pitch Delay)
    % =========================================================================
    
    % 1. UNPACK PARAMETERS
    m = veh_params.m; Iz = veh_params.Iz; lf = veh_params.lf; lr = veh_params.lr; L = veh_params.L;
    tw = veh_params.tw; h_cg = veh_params.h_cg; Rw = veh_params.Rw; Iw = veh_params.Iw; 
    G = veh_params.G; g = veh_params.g; rho = veh_params.rho; CdA = veh_params.CdA;
    roll_bias_f = veh_params.roll_bias_f; mu_max = veh_params.mu_max; C_rr = veh_params.C_rr;
    ks_f = veh_params.ks_f; ks_r = veh_params.ks_r; C_tire = veh_params.C_tire; E_tire = veh_params.E_tire;
    
    if abs(vx) < 0.5, vx_safe = 0.5 * sign(vx + 1e-6); else, vx_safe = vx; end
    F_aero_drag = 0.5 * rho * CdA * vx_safe * abs(vx_safe);

    % ---------------------------------------------------------------------
    % 2. INSTANTANEOUS WEIGHT TRANSFER (QUASI-STATIC)
    % ---------------------------------------------------------------------
    Fx_total_tq = (Trr_m + Trl_m)*G + Trr_f + Trl_f + Tf_f;
    ax_inst = (Fx_total_tq/Rw - F_aero_drag) / m;
    ay_inst = vx_safe * r;
    
    dFz_x = m * ax_inst * (h_cg / L);
    dFz_y = m * ay_inst * (h_cg / tw);
    
    Fz_f_tot = m * g * (lr / L) - dFz_x;
    Fz_r_tot = m * g * (lf / L) + dFz_x;
    
    % Instant distribution based on static roll bias
    Fz_fl = max(100, Fz_f_tot/2 - dFz_y * roll_bias_f);
    Fz_fr = max(100, Fz_f_tot/2 + dFz_y * roll_bias_f);
    Fz_rl = max(100, Fz_r_tot/2 - dFz_y * (1 - roll_bias_f));
    Fz_rr = max(100, Fz_r_tot/2 + dFz_y * (1 - roll_bias_f));
    Fz_vec = [Fz_fl, Fz_fr, Fz_rl, Fz_rr];
    
    % ---------------------------------------------------------------------
    % 3. PACEJKA COMBINED SLIP
    % ---------------------------------------------------------------------
    B_f = ks_f / (C_tire * mu_max * (Fz_f_tot/2 + 1e-6)); 
    B_r = ks_r / (C_tire * mu_max * (Fz_r_tot/2 + 1e-6)); 
    
    v_hub_fl = vx_safe - (tw / 2) * r; v_hub_fr = vx_safe + (tw / 2) * r;
    v_hub_rl = vx_safe - (tw / 2) * r; v_hub_rr = vx_safe + (tw / 2) * r;
    
    k_fl = (w_fl * Rw - v_hub_fl) / max(abs(v_hub_fl), 1.0);
    k_fr = (w_fr * Rw - v_hub_fr) / max(abs(v_hub_fr), 1.0);
    k_rl = (w_rl * Rw - v_hub_rl) / max(abs(v_hub_rl), 1.0);
    k_rr = (w_rr * Rw - v_hub_rr) / max(abs(v_hub_rr), 1.0);
    
    alpha_fl = delta - atan((vy + lf * r) / max(abs(v_hub_fl), 1.0));
    alpha_fr = delta - atan((vy + lf * r) / max(abs(v_hub_fr), 1.0));
    alpha_rl = -atan((vy - lr * r) / max(abs(v_hub_rl), 1.0));
    alpha_rr = -atan((vy - lr * r) / max(abs(v_hub_rr), 1.0));
    
    sigma_fl = sqrt(k_fl^2 + tan(alpha_fl)^2) + 1e-6;
    sigma_fr = sqrt(k_fr^2 + tan(alpha_fr)^2) + 1e-6;
    sigma_rl = sqrt(k_rl^2 + tan(alpha_rl)^2) + 1e-6;
    sigma_rr = sqrt(k_rr^2 + tan(alpha_rr)^2) + 1e-6;
    
    F_tot_fl = mu_max * Fz_fl * sin(C_tire * atan(B_f * sigma_fl - E_tire * (B_f * sigma_fl - atan(B_f * sigma_fl))));
    F_tot_fr = mu_max * Fz_fr * sin(C_tire * atan(B_f * sigma_fr - E_tire * (B_f * sigma_fr - atan(B_f * sigma_fr))));
    F_tot_rl = mu_max * Fz_rl * sin(C_tire * atan(B_r * sigma_rl - E_tire * (B_r * sigma_rl - atan(B_r * sigma_rl))));
    F_tot_rr = mu_max * Fz_rr * sin(C_tire * atan(B_r * sigma_rr - E_tire * (B_r * sigma_rr - atan(B_r * sigma_rr))));
    
    Fx_fl = F_tot_fl * (k_fl / sigma_fl) - C_rr * Fz_fl * tanh(v_hub_fl * 10);
    Fx_fr = F_tot_fr * (k_fr / sigma_fr) - C_rr * Fz_fr * tanh(v_hub_fr * 10);
    Fx_rl = F_tot_rl * (k_rl / sigma_rl) - C_rr * Fz_rl * tanh(v_hub_rl * 10);
    Fx_rr = F_tot_rr * (k_rr / sigma_rr) - C_rr * Fz_rr * tanh(v_hub_rr * 10);
    Fx_vec = [Fx_fl, Fx_fr, Fx_rl, Fx_rr];
    
    Fy_fl = F_tot_fl * (tan(alpha_fl) / sigma_fl);
    Fy_fr = F_tot_fr * (tan(alpha_fr) / sigma_fr);
    Fy_rl = F_tot_rl * (tan(alpha_rl) / sigma_rl);
    Fy_rr = F_tot_rr * (tan(alpha_rr) / sigma_rr);
    Fy_vec = [Fy_fl, Fy_fr, Fy_rl, Fy_rr];
    
    % 4. CHASSIS INTEGRATORS
    w_fl_dot = (-abs(Tf_f/2)*sign(w_fl) - Fx_fl*Rw)/Iw;
    w_fr_dot = (-abs(Tf_f/2)*sign(w_fr) - Fx_fr*Rw)/Iw;
    w_rl_dot = (Trl_m*G - abs(Trl_f)*sign(w_rl) - Fx_rl*Rw)/Iw;
    w_rr_dot = (Trr_m*G - abs(Trr_f)*sign(w_rr) - Fx_rr*Rw)/Iw;
    w_dot_vec = [w_fl_dot, w_fr_dot, w_rl_dot, w_rr_dot];
    w_vec = [w_fl, w_fr, w_rl, w_rr];
    
    sum_Fx = (Fx_fl + Fx_fr)*cos(delta) - (Fy_fl + Fy_fr)*sin(delta) + Fx_rl + Fx_rr;
    vx_dot = (sum_Fx - F_aero_drag)/m + vy*r;
    sum_Fy = (Fy_fl + Fy_fr)*cos(delta) + (Fx_fl + Fx_fr)*sin(delta) + Fy_rl + Fy_rr;
    vy_dot = sum_Fy/m - vx_safe*r;
    
    r_dot = (lf*((Fy_fl + Fy_fr)*cos(delta) + (Fx_fl + Fx_fr)*sin(delta)) - lr*(Fy_rl + Fy_rr) + (Fx_rr - Fx_rl)*(tw/2))/Iz;
    
    X_dot = vx_safe*cos(psi) - vy*sin(psi);
    Y_dot = vx_safe*sin(psi) + vy*cos(psi);
    psi_dot = r; s_dot = vx_safe;
    
    % THERMALS & SOC (Simplified Baseline)
    P_mech = (Trr_m + Trl_m)*G*(vx_safe/Rw);
    I_curr = (P_mech / 0.90) / veh_params.V_pack;
    SOC_dot = -I_curr/(veh_params.Cap_Ah*3600);
    T_batt_dot = ((I_curr^2)*veh_params.R_pack - veh_params.hA_cool_batt*(T_batt-veh_params.T_coolant_batt))/(veh_params.m_batt*veh_params.cp_batt);
    T_mot_dot  = (abs(P_mech*0.1) - veh_params.hA_cool_motor*(T_motor-veh_params.T_ambient))/(veh_params.m_motor*veh_params.cp_motor);
end

== matlab function RLS_1a/Scopes/MATLAB Function ==
  settings: updateMethod=DISCRETE
  data: X_curr input; Y_curr input; psi_curr input; vx_curr input; delta_curr input; t_curr input; X_track parameter; Y_track parameter
function live_track_plotter(X_curr, Y_curr, psi_curr, vx_curr, delta_curr, t_curr, X_track, Y_track)
    coder.extrinsic('figure', 'plot', 'hold', 'axis', 'title', 'xlabel', 'ylabel', 'set', 'drawnow', 'animatedline', 'addpoints', 'legend', 'grid', 'patch', 'text');
    
    persistent hFig hCar hTrail hText counter 
    persistent hTimer1 hTimer2 hTimer3 hTimer4 hTimer5
    persistent lap_count lap_start_time lap_trigger_ready
    persistent past_lap_1 past_lap_2 past_lap_3 past_lap_4 past_lap_5
    
    if isempty(counter)
        counter = 0;
        lap_count = 1;
        lap_start_time = 0;
        lap_trigger_ready = false;
        
        past_lap_1 = 0; past_lap_2 = 0; past_lap_3 = 0; past_lap_4 = 0; past_lap_5 = 0;
        
        hFig = figure('Name', 'Live Telemetry: Silverstone / DLC', 'Color', 'w', 'Position', [100, 100, 800, 600]);
        plot(X_track, Y_track, '--', 'Color', [0.4 0.4 0.4], 'LineWidth', 1.5); hold on;
        
        plot(X_track(1), Y_track(1), 'ko', 'MarkerSize', 10, 'MarkerFaceColor', 'g', 'LineWidth', 1.5);
        text(X_track(1) - 50, Y_track(1) + 70, 'Start / Finish', 'FontSize', 10, 'FontWeight', 'bold', 'Color', 'k', 'BackgroundColor', [1 1 1 0.7]);
        
        hTrail = animatedline('Color', 'b', 'LineWidth', 1.5);
        
        hCar = patch(0, 0, [0.8 0 0], 'EdgeColor', 'k', 'LineWidth', 1);
        set(hCar, 'FaceAlpha', 0.8); 
        
        hText = text(0, 0, ' Init...', 'FontSize', 10, 'FontWeight', 'bold', 'BackgroundColor', [1 1 1 0.8], 'EdgeColor', 'k', 'Margin', 2);
        
        box_props = {'Units', 'normalized', 'HorizontalAlignment', 'right', 'FontSize', 12, 'FontWeight', 'bold', 'BackgroundColor', [1 1 1 0.9], 'EdgeColor', 'k', 'Margin', 4, 'Visible', 'off'};
        
        hTimer1 = text(0.95, 0.95, '', box_props{:});
        hTimer2 = text(0.95, 0.89, '', box_props{:});
        hTimer3 = text(0.95, 0.83, '', box_props{:});
        hTimer4 = text(0.95, 0.77, '', box_props{:});
        hTimer5 = text(0.95, 0.71, '', box_props{:});
        
        axis equal; grid on;
        title('Live Vehicle Tracking with Telemetry');
        xlabel('X Position (meters)'); ylabel('Y Position (meters)');
        legend('Reference Track', 'Start/Finish', 'Driven Path', 'EV Position & Heading', 'Telemetry', 'Location', 'best');
    end
    counter = counter + 1;
    
    dist_to_origin = sqrt((X_curr - X_track(1))^2 + (Y_curr - Y_track(1))^2);
    
    if dist_to_origin > 50
        lap_trigger_ready = true;
    end
    
    if lap_trigger_ready && dist_to_origin < 15
        completed_lap_time = t_curr - lap_start_time;
        if lap_count == 1
            past_lap_1 = completed_lap_time;
        elseif lap_count == 2
            past_lap_2 = completed_lap_time;
        elseif lap_count == 3
            past_lap_3 = completed_lap_time;
        elseif lap_count == 4
            past_lap_4 = completed_lap_time;
        elseif lap_count == 5
            past_lap_5 = completed_lap_time;
        end
        
        lap_count = lap_count + 1;
        lap_start_time = t_curr;
        lap_trigger_ready = false; 
    end
    
    if mod(counter, 10) == 0
        addpoints(hTrail, X_curr, Y_curr);
        
        % --- REALISTIC 1:1 VEHICLE SCALING ---
        L_vis = 4.5; % 4.5 meters long
        W_vis = 1.9; % 1.9 meters wide
        % ------------------------------------
        
        base_X = [L_vis/2,  L_vis*0.3,   0,       -L_vis*0.35, -L_vis/2,  -L_vis/2,   -L_vis*0.35,  0,        L_vis*0.3,   L_vis/2];
        base_Y = [0,        W_vis*0.45, W_vis/2,  W_vis/2,     W_vis*0.3, -W_vis*0.3, -W_vis/2,    -W_vis/2, -W_vis*0.45, 0];
        
        R = [cos(psi_curr), -sin(psi_curr); 
             sin(psi_curr),  cos(psi_curr)];
             
        rotated_coords = R * [base_X; base_Y];
        final_X = rotated_coords(1, :) + X_curr;
        final_Y = rotated_coords(2, :) + Y_curr;
        
        set(hCar, 'XData', final_X, 'YData', final_Y);
        
        speed_kmh = vx_curr * 3.6;
        steer_deg = delta_curr * (180 / pi);
        
        telemetry_str = sprintf(' Spd: %.1f km/h\n Steer. Ang.: %.1f deg', speed_kmh, steer_deg);
        
        % Brought the text box much closer to the scaled vehicle
        set(hText, 'Position', [X_curr + 10, Y_curr + 10], 'String', telemetry_str);
        
        current_live_time = t_curr - lap_start_time;
        
        if lap_count == 1
            set(hTimer1, 'String', sprintf(' Lap 1: %d:%06.3f (Live) ', int32(floor(current_live_time/60)), mod(current_live_time, 60)), 'Visible', 'on');
        elseif lap_count > 1
            set(hTimer1, 'String', sprintf(' Lap 1: %d:%06.3f ', int32(floor(past_lap_1/60)), mod(past_lap_1, 60)), 'Visible', 'on');
        end
        
        if lap_count == 2
            set(hTimer2, 'String', sprintf(' Lap 2: %d:%06.3f (Live) ', int32(floor(current_live_time/60)), mod(current_live_time, 60)), 'Visible', 'on');
        elseif lap_count > 2
            set(hTimer2, 'String', sprintf(' Lap 2: %d:%06.3f ', int32(floor(past_lap_2/60)), mod(past_lap_2, 60)), 'Visible', 'on');
        end
        
        if lap_count == 3
            set(hTimer3, 'String', sprintf(' Lap 3: %d:%06.3f (Live) ', int32(floor(current_live_time/60)), mod(current_live_time, 60)), 'Visible', 'on');
        elseif lap_count > 3
            set(hTimer3, 'String', sprintf(' Lap 3: %d:%06.3f ', int32(floor(past_lap_3/60)), mod(past_lap_3, 60)), 'Visible', 'on');
        end
        
        if lap_count == 4
            set(hTimer4, 'String', sprintf(' Lap 4: %d:%06.3f (Live) ', int32(floor(current_live_time/60)), mod(current_live_time, 60)), 'Visible', 'on');
        elseif lap_count > 4
            set(hTimer4, 'String', sprintf(' Lap 4: %d:%06.3f ', int32(floor(past_lap_4/60)), mod(past_lap_4, 60)), 'Visible', 'on');
        end
        
        if lap_count == 5
            set(hTimer5, 'String', sprintf(' Lap 5: %d:%06.3f (Live) ', int32(floor(current_live_time/60)), mod(current_live_time, 60)), 'Visible', 'on');
        elseif lap_count > 5
            set(hTimer5, 'String', sprintf(' Lap 5: %d:%06.3f ', int32(floor(past_lap_5/60)), mod(past_lap_5, 60)), 'Visible', 'on');
        end
        
        drawnow limitrate; 
    end
end

== matlab function RLS_1a/Scopes/MATLAB Function1 ==
  settings: updateMethod=DISCRETE
  data: delta input; psi input; psi_ref input; Fx input; Fy input; Fz input; Trl input; Trr input; Tf_f input; Trl_f input; Trr_f input; w_vec input
function vehicle_frame_plotter(delta, psi, psi_ref, Fx, Fy, Fz, Trl, Trr, Tf_f, Trl_f, Trr_f, w_vec)
    coder.extrinsic('figure', 'plot', 'hold', 'axis', 'title', 'set', 'drawnow', 'patch', 'text', 'line', 'quiver', 'sprintf');
    
    persistent hFig hWheels hSteer hSpokes hPsiRef hPsiAct hFlags hTqFlags hMotors hAxle hCircles hGdots hSwLabel hRwLabel counter
    
    if isempty(counter)
        counter = 0;
        hWheels = zeros(1,4); hFlags = zeros(1,4); hTqFlags = zeros(1,2);
        hMotors = zeros(1,2); hSpokes = zeros(1,3); hCircles = zeros(1,4); hGdots = zeros(1,4);
        hSwLabel = 0.0; hRwLabel = 0.0;
        
        hFig = figure('Name', 'Vehicle Frame Telemetry', 'Color', 'w', 'Position', [950, 100, 750, 750]);
        hold on;
        
        plot([-1, 1, 1, -1, -1], [2, 2, -2, -2, 2], 'k', 'LineWidth', 2);
        hAxle = line([1, -1], [1.5, 1.5], 'Color', [0.2 0.2 0.2], 'LineWidth', 2);
        
        wheel_base = [-.2, .2, .2, -.2]; wheel_wid = [.4, .4, -.4, -.4];
        for i = 1:4; hWheels(i) = double(patch(0, 0, [0.3 0.3 0.3])); end
        
        m_b = [-.15, .15, .15, -.15]; m_w = [.2, .2, -.2, -.2];
        hMotors(1) = double(patch(m_b + 0.6, m_w - 1.5, [0.5 0.5 0.5]));
        hMotors(2) = double(patch(m_b - 0.6, m_w - 1.5, [0.5 0.5 0.5]));
        
        th_c = 0:0.1:2*pi;
        circle_x = cos(th_c); circle_y = sin(th_c);
        c_pos = [2.0, 2.3; -2.0, 2.3; 2.0, -2.3; -2.0, -2.3];
        for i = 1:4
            hCircles(i) = double(plot(c_pos(i,1) + 0.5*circle_x, c_pos(i,2) + 0.5*circle_y, 'Color', [0.6 0 0.6], 'LineStyle', '--', 'LineWidth', 1.2));
            hGdots(i) = double(plot(c_pos(i,1), c_pos(i,2), 'mo', 'MarkerFaceColor', 'm', 'MarkerSize', 5));
        end
        
        th = 0:0.1:2*pi;
        hSteer = double(plot(0.4*cos(th), 0.4*sin(th) + 0.5, 'k', 'LineWidth', 3));
        hSpokes(1) = double(line([0, 0], [0.5, 0.5], 'Color', 'k', 'LineWidth', 2.5));
        hSpokes(2) = double(line([0, 0], [0.5, 0.5], 'Color', 'k', 'LineWidth', 2.5));
        hSpokes(3) = double(line([0, 0], [0.5, 0.5], 'Color', 'k', 'LineWidth', 2.5));
        
        hPsiRef = double(quiver(0, 1.8, 0, 0.8, 'r', 'LineWidth', 2.5, 'MaxHeadSize', 2));
        hPsiAct = double(quiver(0, 1.8, 0, 0.8, 'b', 'LineWidth', 2.5, 'MaxHeadSize', 2));
        
        for i = 1:4; hFlags(i) = double(text(0, 0, '', 'FontSize', 8, 'BackgroundColor', [1 1 1 0.8], 'EdgeColor', 'k')); end
        hTqFlags(1) = double(text(0.6, -1.1, '', 'FontSize', 8, 'FontWeight', 'bold', 'HorizontalAlignment', 'center'));
        hTqFlags(2) = double(text(-0.6, -1.1, '', 'FontSize', 8, 'FontWeight', 'bold', 'HorizontalAlignment', 'center'));
        
        hSwLabel = double(text(0, 0, '', 'FontSize', 9, 'FontWeight', 'bold', 'HorizontalAlignment', 'center'));
        hRwLabel = double(text(0, 2.3, '', 'FontSize', 9, 'FontWeight', 'bold', 'HorizontalAlignment', 'center', 'Color', [0 0.5 0]));
        
        axis([-4.5 4.5 -4.5 4.5]); axis equal; grid on;
        title('Dynamics: Forces, Steering & Friction Circles');
    end
    counter = counter + 1;
    if mod(counter, 10) == 0
        R_delta = [cos(delta) -sin(delta); sin(delta) cos(delta)];
        w_orig = [-.2 .2 .2 -.2; .4 .4 -.4 -.4]; 
        w_rot = R_delta * w_orig;
        
        set(hWheels(1), 'XData', w_rot(1,:) + 1, 'YData', w_rot(2,:) + 1.5);
        set(hWheels(2), 'XData', w_rot(1,:) - 1, 'YData', w_rot(2,:) + 1.5);
        set(hWheels(3), 'XData', w_orig(1,:) + 1, 'YData', w_orig(2,:) - 1.5);
        set(hWheels(4), 'XData', w_orig(1,:) - 1, 'YData', w_orig(2,:) - 1.5);
        
        set(hAxle, 'XData', [mean(w_rot(1,:) + 1), mean(w_rot(1,:) - 1)], 'YData', [mean(w_rot(2,:) + 1.5), mean(w_rot(2,:) + 1.5)]);
        
        sw_a = delta * 14; 
        th_sw = (0:0.1:2*pi) + sw_a;
        set(hSteer, 'XData', 0.4*cos(th_sw), 'YData', 0.4*sin(th_sw) + 0.5);
        
        spk = [0, pi, 1.5*pi] + sw_a;
        for j=1:3; set(hSpokes(j), 'XData', [0, 0.4*cos(spk(j))], 'YData', [0.5, 0.5 + 0.4*sin(spk(j))]); end
        
        set(hSwLabel, 'Position', [0, 0.5], 'String', sprintf('SW: %.1f deg', sw_a * 180/pi));
        set(hRwLabel, 'String', sprintf('RW: %.1f deg', delta * 180/pi));
        
        psi_e = psi_ref - psi; 
        set(hPsiRef, 'UData', 0.8*sin(psi_e), 'VData', 0.8*cos(psi_e));
        set(hPsiAct, 'UData', 0, 'VData', 0.8);
        
        fb = [abs(Tf_f/2), abs(Tf_f/2), abs(Trl_f), abs(Trr_f)]; mu = 1.0;
        c_pos = [2.0, 2.3; -2.0, 2.3; 2.0, -2.3; -2.0, -2.3];
        th_c = 0:0.1:2*pi;
        
        % Convert rad/s to RPM
        rpm_vec = w_vec * (30 / pi);
        
        for i = 1:4
            if fb(i) > 5; set(hWheels(i), 'FaceColor', [0.8 0 0]); else set(hWheels(i), 'FaceColor', [0.3 0.3 0.3]); end
            F_max = max(100, mu * Fz(i));
            scale = 0.5 / 6000; 
            set(hCircles(i), 'XData', c_pos(i,1) + F_max*scale*cos(th_c), 'YData', c_pos(i,2) + F_max*scale*sin(th_c));
            set(hGdots(i), 'XData', c_pos(i,1) + Fy(i)*scale, 'YData', c_pos(i,2) + Fx(i)*scale);
        end
        
        mt = [Trl, Trr];
        for k = 1:2
            if mt(k) > 0.1; set(hMotors(k), 'FaceColor', [0 0.7 0]); elseif mt(k) < -0.1; set(hMotors(k), 'FaceColor', [0.7 0 0]); else set(hMotors(k), 'FaceColor', [0.5 0.5 0.5]); end
            set(hTqFlags(k), 'String', sprintf('Mot. Trq.\n%.1f Nm', mt(k)));
        end
        
        pos = [2.8, 1.5; -4.1, 1.5; 2.8, -1.5; -4.1, -1.5];
        for i = 1:4
            f_str = sprintf('Fx: %.0f\nFy: %.0f\nFz: %.0f\nFric: %.1f\nRPM: %.0f', Fx(i), Fy(i), Fz(i), fb(i), rpm_vec(i));
            set(hFlags(i), 'Position', [pos(i,1), pos(i,2)], 'String', f_str);
        end
        drawnow limitrate;
    end
end
